simulink model "test_quadcopter"  (R2021b)
settings: Solver=ode45  StartTime=0.0  StopTime=300  FixedStep=Ts  MaxStep=0.001  RelTol=1e-3  AbsTol=1e-3
model workspace (MATLAB code in the model file):
  | load('xy_data_membrane.mat');
undefined symbols (not defined in the file): kd_altitude, kd_attitude, kd_position, ki_altitude, ki_attitude, kp_altitude, kp_attitude, kp_position, propeller, X, x0, xrot, Y, y0, yrot, Z, z0, zrot
libraries: sm_lib x83, fl_lib x40, nesl_utility x34, aerolibwind2 x6, slpidlib x4
(part 4 of 4)

== system test_quadcopter/Quadcopter Model and Control/Motor Propeller 2/Propeller Thrust Calculator ==
  Air Density : fl_lib/Physical Signals/Sources/PS Constant  constant=1.225 kg/m^3
  PS Gain : fl_lib/Physical Signals/Functions/PS Gain  gain=1/60
  PS Math Function : fl_lib/Physical Signals/Functions/PS Math Function  fcn_choice=foundation.enum.math_function.pow  v=4
      settings: SourceProductBaseCode=SS
  PS Math Function1 : fl_lib/Physical Signals/Functions/PS Math Function  fcn_choice=foundation.enum.math_function.square  v=2
      settings: SourceProductBaseCode=SS
  PS Product : fl_lib/Physical Signals/Functions/PS Product
  PS Product1 : fl_lib/Physical Signals/Functions/PS Product
  PS Product2 : fl_lib/Physical Signals/Functions/PS Product
  Propeller Diameter : fl_lib/Physical Signals/Sources/PS Constant  constant=propeller.diameter m
  Ct : PMIOPort  Side=Left
  Propeller Speed : PMIOPort  Port=2  Side=Left
  Thrust : PMIOPort  Port=3  Side=Right
  connections:
  PS Math Function/LConn1 -- Propeller Diameter/RConn1
  PS Math Function1/RConn1 -- PS Product1/LConn1
  Air Density/RConn1 -- PS Product1/LConn2
  PS Product1/RConn1 -- PS Product2/LConn2
  PS Gain/RConn1 -- PS Math Function1/LConn1
  PS Math Function/RConn1 -- PS Product/LConn2
  PS Product/RConn1 -- PS Product2/LConn1
  Propeller Speed/RConn1 -- PS Gain/LConn1
  Thrust/RConn1 -- PS Product2/RConn1
  PS Product/LConn1 -- Ct/RConn1

== system test_quadcopter/Quadcopter Model and Control/Motor Propeller 2/Thrust Coefficient Calculator ==
  m/s : Inport
  Add : Sum  Inputs=+++
  Constant : Constant  Value=0.1072
  Gain1 : Gain  Gain=-0.008716
  Gain4 : Gain  Gain=-0.001589
  Math Function : Math  Operator=square  SaturateOnIntegerOverflow=on
  Simulink-PS Converter : nesl_utility/Simulink-PS Converter  PhysicalDomain=network_engine_domain  SubClassName=ps_input  LeftPortType=input  RightPortType=output  PseudoPeriodic=off  Frequencies=[]  NoiseDistribution=none  NoiseParameters=[]  Unit=1/(rev^2)  AffineConversion=off  FilteringAndDerivatives=provide  SimscapeFilterOrder=1  InputFilterTimeConstant=0.001  UdotUserProvided=0
      settings: SourceProductBaseCode=PW,SS
  Ct : PMIOPort  Side=Right
  wires:
  Math Function/1 -> Gain4/1
  m/s/1 -> Gain1/1, Math Function/1
  Add/1 -> Simulink-PS Converter/1
  Gain4/1 -> Add/1
  Gain1/1 -> Add/2
  Constant/1 -> Add/3
  connections:
  Simulink-PS Converter/RConn1 -- Ct/RConn1

== system test_quadcopter/Quadcopter Model and Control/Motor Propeller 3 /Propeller Thrust Calculator ==
  Air Density : fl_lib/Physical Signals/Sources/PS Constant  constant=1.225 kg/m^3
  PS Gain : fl_lib/Physical Signals/Functions/PS Gain  gain=1/60
  PS Math Function : fl_lib/Physical Signals/Functions/PS Math Function  fcn_choice=foundation.enum.math_function.pow  v=4
      settings: SourceProductBaseCode=SS
  PS Math Function1 : fl_lib/Physical Signals/Functions/PS Math Function  fcn_choice=foundation.enum.math_function.square  v=2
      settings: SourceProductBaseCode=SS
  PS Product : fl_lib/Physical Signals/Functions/PS Product
  PS Product1 : fl_lib/Physical Signals/Functions/PS Product
  PS Product2 : fl_lib/Physical Signals/Functions/PS Product
  Propeller Diameter : fl_lib/Physical Signals/Sources/PS Constant  constant=propeller.diameter m
  Ct : PMIOPort  Side=Left
  Propeller Speed : PMIOPort  Port=2  Side=Left
  Thrust : PMIOPort  Port=3  Side=Right
  connections:
  PS Math Function/LConn1 -- Propeller Diameter/RConn1
  PS Math Function1/RConn1 -- PS Product1/LConn1
  Air Density/RConn1 -- PS Product1/LConn2
  PS Product1/RConn1 -- PS Product2/LConn2
  PS Math Function/RConn1 -- PS Product/LConn2
  PS Product/RConn1 -- PS Product2/LConn1
  PS Math Function1/LConn1 -- PS Gain/RConn1
  Propeller Speed/RConn1 -- PS Gain/LConn1
  Thrust/RConn1 -- PS Product2/RConn1
  PS Product/LConn1 -- Ct/RConn1

== system test_quadcopter/Quadcopter Model and Control/Motor Propeller 3 /Thrust Coefficient Calculator ==
  m/s : Inport
  Add : Sum  Inputs=+++
  Constant : Constant  Value=0.1072
  Gain1 : Gain  Gain=-0.008716
  Gain4 : Gain  Gain=-0.001589
  Math Function : Math  Operator=square  SaturateOnIntegerOverflow=on
  Simulink-PS Converter : nesl_utility/Simulink-PS Converter  PhysicalDomain=network_engine_domain  SubClassName=ps_input  LeftPortType=input  RightPortType=output  PseudoPeriodic=off  Frequencies=[]  NoiseDistribution=none  NoiseParameters=[]  Unit=1/(rev)^2  AffineConversion=off  FilteringAndDerivatives=provide  SimscapeFilterOrder=1  InputFilterTimeConstant=0.001  UdotUserProvided=0
      settings: SourceProductBaseCode=PW,SS
  Ct : PMIOPort  Side=Right
  wires:
  Constant/1 -> Add/3
  Gain4/1 -> Add/1
  Add/1 -> Simulink-PS Converter/1
  m/s/1 -> Gain1/1, Math Function/1
  Math Function/1 -> Gain4/1
  Gain1/1 -> Add/2
  connections:
  Simulink-PS Converter/RConn1 -- Ct/RConn1

== system test_quadcopter/Quadcopter Model and Control/Motor Propeller 4/Propeller Thrust Calculator ==
  Air Density : fl_lib/Physical Signals/Sources/PS Constant  constant=1.225 kg/m^3
  PS Gain : fl_lib/Physical Signals/Functions/PS Gain  gain=1/60
  PS Math Function : fl_lib/Physical Signals/Functions/PS Math Function  fcn_choice=foundation.enum.math_function.pow  v=4
      settings: SourceProductBaseCode=SS
  PS Math Function1 : fl_lib/Physical Signals/Functions/PS Math Function  fcn_choice=foundation.enum.math_function.square  v=2
      settings: SourceProductBaseCode=SS
  PS Product : fl_lib/Physical Signals/Functions/PS Product
  PS Product1 : fl_lib/Physical Signals/Functions/PS Product
  PS Product2 : fl_lib/Physical Signals/Functions/PS Product
  Propeller Diameter : fl_lib/Physical Signals/Sources/PS Constant  constant=propeller.diameter m
  Ct : PMIOPort  Side=Left
  Propeller Speed : PMIOPort  Port=2  Side=Left
  Thrust : PMIOPort  Port=3  Side=Right
  connections:
  PS Math Function/LConn1 -- Propeller Diameter/RConn1
  PS Math Function1/RConn1 -- PS Product1/LConn1
  Air Density/RConn1 -- PS Product1/LConn2
  PS Product1/RConn1 -- PS Product2/LConn2
  PS Gain/RConn1 -- PS Math Function1/LConn1
  PS Math Function/RConn1 -- PS Product/LConn2
  PS Product/RConn1 -- PS Product2/LConn1
  Propeller Speed/RConn1 -- PS Gain/LConn1
  Thrust/RConn1 -- PS Product2/RConn1
  PS Product/LConn1 -- Ct/RConn1

== system test_quadcopter/Quadcopter Model and Control/Motor Propeller 4/Thrust Coefficient Calculator ==
  m/s : Inport
  Add : Sum  Inputs=+++
  Constant : Constant  Value=0.1072
  Gain1 : Gain  Gain=-0.008716
  Gain4 : Gain  Gain=-0.001589
  Math Function : Math  Operator=square  SaturateOnIntegerOverflow=on
  Simulink-PS Converter : nesl_utility/Simulink-PS Converter  PhysicalDomain=network_engine_domain  SubClassName=ps_input  LeftPortType=input  RightPortType=output  PseudoPeriodic=off  Frequencies=[]  NoiseDistribution=none  NoiseParameters=[]  Unit=1/(rev)^2  AffineConversion=off  FilteringAndDerivatives=provide  SimscapeFilterOrder=1  InputFilterTimeConstant=0.001  UdotUserProvided=0
      settings: SourceProductBaseCode=PW,SS
  Ct : PMIOPort  Side=Right
  wires:
  Constant/1 -> Add/3
  Gain4/1 -> Add/1
  Add/1 -> Simulink-PS Converter/1
  m/s/1 -> Gain1/1, Math Function/1
  Math Function/1 -> Gain4/1
  Gain1/1 -> Add/2
  connections:
  Simulink-PS Converter/RConn1 -- Ct/RConn1

== matlab function test_quadcopter/Flight and Trajectory Generation /Trajectory Generator1 ==
  settings: updateMethod=DISCRETE
  data: pos_des output; vel_des output; yaw_des output; homePose input
 function [pos_des,vel_des,yaw_des]  = trajectory_generator(homePose)
%% Altitude generator
X0 = homePose(1,1);
Y0 = homePose(2,1);
Z0 = homePose(3,1);
Xf = X0;
Yf = Y0;
Zf = 5 + Z0;
pos_des = [Xf;Yf;Zf];
vel_des = [2;2;2];
yaw_des = 0;

== matlab function test_quadcopter/Flight and Trajectory Generation /Position Controller/Roll Pitch Yaw Controller/Direction Cosine Matrix ==
  data: RPY input; DCM output
function DCM = fcn(RPY)


% Euler Angles
phi = RPY(1);
theta = RPY(2);
psi = RPY(3);

DCM = [cos(theta)*cos(psi) cos(theta)*sin(psi) -sin(theta);  
    -cos(phi)*sin(psi)+sin(phi)*sin(theta)*cos(psi) cos(phi)*cos(psi)+sin(phi)*sin(theta)*sin(psi) sin(phi)*cos(theta);
    sin(phi)*sin(psi)+cos(phi)*sin(theta)*cos(psi) -sin(phi)*cos(psi)+cos(phi)*sin(theta)*sin(psi) cos(phi)*cos(theta)];

end

== matlab function test_quadcopter/Quadcopter Model and Control/Quadcopter Chassis/Quaternion to Euler Angles Conversion1 ==
  data: Quaternion input; roll output; pitch output; yaw output
function [roll,pitch,yaw] = quaternion_to_euler_angles_conversion(Quaternion)
% This MATLAB function converts the quaternions to the Euler Angles

w = Quaternion(1,1);
x = Quaternion(2,1);
y = Quaternion(3,1);
z = Quaternion(4,1);

% roll (x-axis rotation)
sinr_cosp = 2 * (w * x + y * z);
cosr_cosp = 1 - 2 * (x * x + y * y);
roll = atan2(sinr_cosp, cosr_cosp);

% pitch (y-axis rotation)
sinp = 2 * (w * y - z * x);
pitch = asin(sinp);

% yaw (z-axis rotation)
siny_cosp = 2 * (w * z + x * y);
cosy_cosp = 1 - 2 * (y * y + z * z);
yaw = atan2(siny_cosp, cosy_cosp);

end

== matlab function test_quadcopter/Flight and Trajectory Generation /Position Controller/Position Controller1 ==
  data: des_pos input; des_vel input; des_yaw input; pos input; vel input; pitch_des output; roll_des output; yaw_des output; attitude input; kp_position input; kd_position input; DCM output
function [pitch_des,roll_des,yaw_des,DCM] = position_controller(des_pos,des_vel,des_yaw,pos,vel,attitude, kp_position, kd_position)
% This MATLAB function computes the desired roll, pitch and yaw angles to
% control the position of the quadcopter.

% Euler Angles
phi = attitude(1);
theta = attitude(2);
psi = attitude(3);

%% Obtain the desired state

% Direction Cosine Matrix
DCM = [cos(theta)*cos(psi)                                    cos(theta)*sin(psi)                          -sin(theta);  %% Direction Cosine for Ground
    -cos(phi)*sin(psi)+sin(phi)*sin(theta)*cos(psi) cos(phi)*cos(psi)+sin(phi)*sin(theta)*sin(psi) sin(phi)*cos(theta)
    sin(phi)*sin(psi)+cos(phi)*sin(theta)*cos(psi) -sin(phi)*cos(psi)+cos(phi)*sin(theta)*sin(psi) cos(phi)*cos(theta)];

% Desired Velocity
v_des = DCM*((des_vel - vel) + kp_position*(des_pos - pos));

% Desired Roll, Pitch and Yaw
pitch_des   = (1/(9.81))*(kd_position*v_des(1)); 
roll_des   = (-1/(9.81))*(kd_position*v_des(2)); 
yaw_des = des_yaw;
end
